simulink model "MeshNetwork_4Node_BaseStation"  (R2024b)
settings: Solver=FixedStepAuto  StartTime=0.0  StopTime=210  FixedStep=1  RelTol=1e-3
settings Model: Creator=ARYA MGC  LastModifiedBy=ARYA MGC

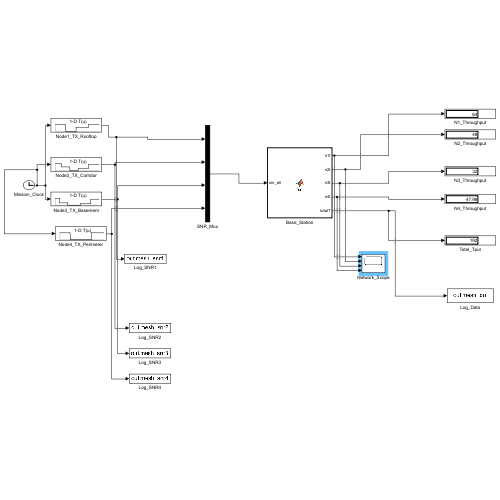
[thumbnail: Simulink's stored preview of the top-level diagram]
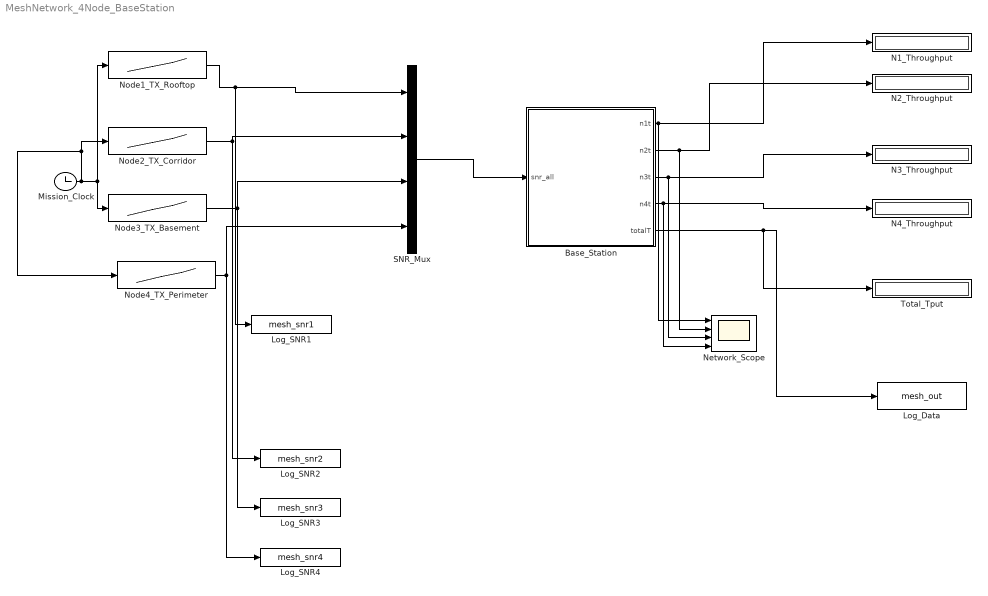
== system MeshNetwork_4Node_BaseStation ==
  Base_Station : MATLAB Function  TreatAsAtomicUnit=on
  Log_Data : ToWorkspace  VariableName=mesh_out  SampleTime=-1
  Log_SNR1 : ToWorkspace  VariableName=mesh_snr1  SampleTime=-1
  Log_SNR2 : ToWorkspace  VariableName=mesh_snr2  SampleTime=-1
  Log_SNR3 : ToWorkspace  VariableName=mesh_snr3  SampleTime=-1
  Log_SNR4 : ToWorkspace  VariableName=mesh_snr4  SampleTime=-1
  Mission_Clock : Clock
  N1_Throughput : Display
  N2_Throughput : Display
  N3_Throughput : Display
  N4_Throughput : Display
  Network_Scope : Scope  NumInputPorts=4
  Node1_TX_Rooftop : Lookup_n-D  NumberOfTableDimensions=1  BreakpointsForDimension1=[0 50 51 100 101 160 161 210]  Table="[30 30 18 18  25  25  30  30]"  InternalRulePriority=Speed  RndMeth=Simplest
  Node2_TX_Corridor : Lookup_n-D  NumberOfTableDimensions=1  BreakpointsForDimension1=[0 30 31 70 71 110 111 160 161 210]  Table="[22 22 15 15 8   8   12  12  20  20]"  InternalRulePriority=Speed  RndMeth=Simplest
  Node3_TX_Basement : Lookup_n-D  NumberOfTableDimensions=1  BreakpointsForDimension1=[0 20 21 60 61 120 121 170 171 210]  Table="[20 20 10 10 5   5   8   8   18  18]"  InternalRulePriority=Speed  RndMeth=Simplest
  Node4_TX_Perimeter : Lookup_n-D  NumberOfTableDimensions=1  BreakpointsForDimension1=[0 50 51 150 151 210]  Table="[25 25 20 20  25  25]"  InternalRulePriority=Speed  RndMeth=Simplest
  SNR_Mux : Mux
  Total_Tput : Display
  wires:
  Mission_Clock/1 -> Node2_TX_Corridor/1, Node4_TX_Perimeter/1, Node1_TX_Rooftop/1, Node3_TX_Basement/1
  Node1_TX_Rooftop/1 -> Log_SNR1/1, SNR_Mux/1
  Node2_TX_Corridor/1 -> SNR_Mux/2, Log_SNR2/1
  Node3_TX_Basement/1 -> Log_SNR3/1, SNR_Mux/3
  Node4_TX_Perimeter/1 -> SNR_Mux/4, Log_SNR4/1
  SNR_Mux/1 -> Base_Station/1(snr_all)
  Base_Station/1(n1t) -> N1_Throughput/1, Network_Scope/1
  Base_Station/2(n2t) -> N2_Throughput/1, Network_Scope/2
  Base_Station/3(n3t) -> N3_Throughput/1, Network_Scope/3
  Base_Station/4(n4t) -> N4_Throughput/1, Network_Scope/4
  Base_Station/5(totalT) -> Total_Tput/1, Log_Data/1

== matlab function MeshNetwork_4Node_BaseStation/Base_Station ==
  data: snr_all input; n1t output; n2t output; n3t output; n4t output; totalT output
function [n1t, n2t, n3t, n4t, totalT] = fcn(snr_all)
%% BASE STATION - 4 Node Mesh Receiver & Router
coder.extrinsic('process_mesh_nodes');
n1t=0; n2t=0; n3t=0; n4t=0; totalT=0;
[n1t, n2t, n3t, n4t, totalT] = process_mesh_nodes(snr_all);
